simulink model "DMC"  (R2015b)
settings: Solver=VariableStepAuto  StartTime=0.0  StopTime=10.0  RelTol=1e-3
values from neighbouring files (symbols this model uses):
  b = 0.3    [demo_DMC.m]
  m = 1    [demo_DMC.m]
libraries: simulink x2
settings Model: Creator=mgreiff  LastModifiedBy=mgreiff

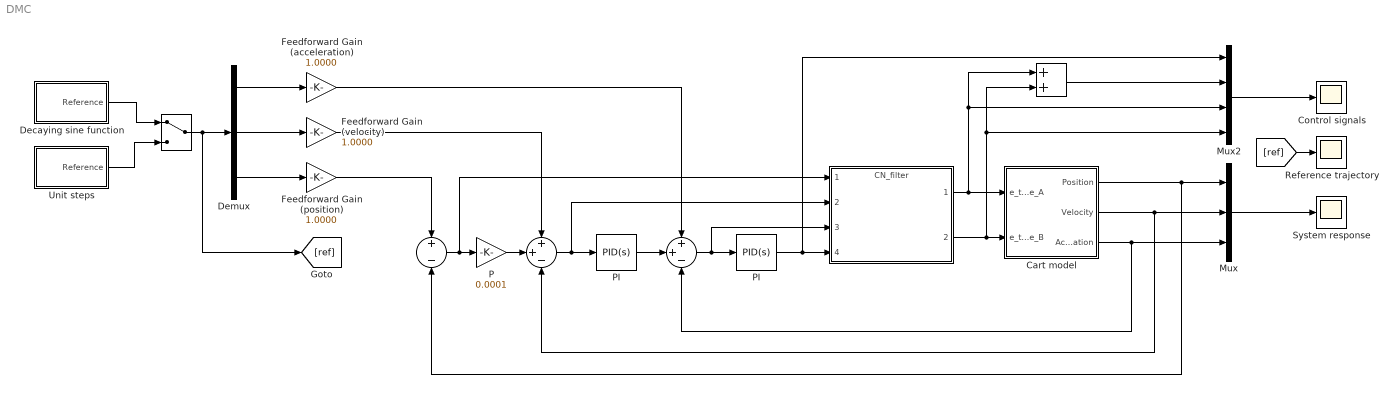
== system DMC ==
  " " : ModelReference  ModelNameDialog=CN_filter.slx  SimulationMode=Normal  ModelReferenceVersion=1.9  CopyOfModelName=CN_filter.slx
  "  " : Sum
  "   " : ManualSwitch
  "        " : Sum  Inputs=++-
  "         " : Sum  Inputs=++-
  "           " : Sum  Inputs=+|-
  "  PI    " : simulink/Continuous/PID Controller  Controller=PID  TimeDomain=Continuous-time  SampleTime=-1  IntegratorMethod=Forward Euler  FilterMethod=Forward Euler  Form=Parallel  UseFilter=on  ControllerParametersSource=internal  P=5  I=0.1  D=0  N=100  InitialConditionSource=internal  InitialConditionForIntegrator=0  InitialConditionForFilter=0  ExternalReset=none  LimitOutput=off  UpperSaturationLimit=inf  LowerSaturationLimit=-inf  LinearizeAsGain=on  AntiWindupMode=none  Kb=1  TrackingMode=off  Kt=1  PParamMin=[]  PParamMax=[]  IParamMin=[]  IParamMax=[]  DParamMin=[]  DParamMax=[]  NParamMin=[]  NParamMax=[]  KbParamMin=[]  KbParamMax=[]  KtParamMin=[]  KtParamMax=[]  POutMin=[]  POutMax=[]  IOutMin=[]  IOutMax=[]  DOutMin=[]  DOutMax=[]  NOutMin=[]  NOutMax=[]  KbOutMin=[]  KbOutMax=[]  KtOutMin=[]  KtOutMax=[]  IntegratorOutMin=[]  IntegratorOutMax=[]  FilterOutMin=[]  FilterOutMax=[]  SumOutMin=[]  SumOutMax=[]  SumI1OutMin=[]  SumI1OutMax=[]  SumI2OutMin=[]  SumI2OutMax=[]  SumI3OutMin=[]  SumI3OutMax=[]  SumDOutMin=[]  SumDOutMax=[]  SaturationOutMin=[]  SaturationOutMax=[]  IntegratorContinuousStateAttributes=''  IntegratorStateMustResolveToSignalObject=off  IntegratorRTWStateStorageClass=Auto  FilterContinuousStateAttributes=''  FilterStateMustResolveToSignalObject=off  FilterRTWStateStorageClass=Auto  DifferentiatorICPrevScaledInput=0  DifferentiatorOutMin=[]  DifferentiatorOutMax=[]
  Cart model : Subsystem
  Control signals : Scope
  Decaying sine function : Subsystem
  Demux : Demux  Outputs=3
  Feedforward Gain (acceleration) : Gain  Gain=1.0000
  Feedforward Gain (position) : Gain  Gain=1.0000
  Feedforward Gain (velocity) : Gain  Gain=1.0000
  Mux : Mux  Inputs=3
  Mux2 : Mux
  P : Gain  Gain=0.0001
  PI : simulink/Continuous/PID Controller  Controller=PID  TimeDomain=Continuous-time  SampleTime=-1  IntegratorMethod=Forward Euler  FilterMethod=Forward Euler  Form=Parallel  UseFilter=on  ControllerParametersSource=internal  P=4  I=0.1  D=0  N=100  InitialConditionSource=internal  InitialConditionForIntegrator=0  InitialConditionForFilter=0  ExternalReset=none  LimitOutput=off  UpperSaturationLimit=inf  LowerSaturationLimit=-inf  LinearizeAsGain=on  AntiWindupMode=none  Kb=1  TrackingMode=off  Kt=1  PParamMin=[]  PParamMax=[]  IParamMin=[]  IParamMax=[]  DParamMin=[]  DParamMax=[]  NParamMin=[]  NParamMax=[]  KbParamMin=[]  KbParamMax=[]  KtParamMin=[]  KtParamMax=[]  POutMin=[]  POutMax=[]  IOutMin=[]  IOutMax=[]  DOutMin=[]  DOutMax=[]  NOutMin=[]  NOutMax=[]  KbOutMin=[]  KbOutMax=[]  KtOutMin=[]  KtOutMax=[]  IntegratorOutMin=[]  IntegratorOutMax=[]  FilterOutMin=[]  FilterOutMax=[]  SumOutMin=[]  SumOutMax=[]  SumI1OutMin=[]  SumI1OutMax=[]  SumI2OutMin=[]  SumI2OutMax=[]  SumI3OutMin=[]  SumI3OutMax=[]  SumDOutMin=[]  SumDOutMax=[]  SaturationOutMin=[]  SaturationOutMax=[]  IntegratorContinuousStateAttributes=''  IntegratorStateMustResolveToSignalObject=off  IntegratorRTWStateStorageClass=Auto  FilterContinuousStateAttributes=''  FilterStateMustResolveToSignalObject=off  FilterRTWStateStorageClass=Auto  DifferentiatorICPrevScaledInput=0  DifferentiatorOutMin=[]  DifferentiatorOutMax=[]
  Reference trajectory : Scope
  System response : Scope
  Unit steps : Subsystem
  wires:
  Cart model/1(Position) -> Mux/1, "           "/2
  Cart model/2(Velocity) -> "        "/3, Mux/2
  " "/1 -> "  "/1, Mux2/3, Cart model/1(e_torque_A)
  " "/2 -> "  "/2, Mux2/4, Cart model/2(e_torque_B)
  "   "/1 -> [ref], Demux/1
  Demux/3 -> Feedforward Gain (position)/1
  "           "/1 -> " "/1, P/1
  P/1 -> "        "/2
  "        "/1 -> "  PI    "/1, " "/2
  "         "/1 -> " "/3, PI/1
  "  PI    "/1 -> "         "/2
  Cart model/3(Acceleration) -> "         "/3, Mux/3
  Demux/2 -> Feedforward Gain (velocity)/1
  Demux/1 -> Feedforward Gain (acceleration)/1
  PI/1 -> Mux2/1, " "/4
  Mux/1 -> System response/1
  Unit steps/1(Reference) -> "   "/2
  Decaying sine function/1(Reference) -> "   "/1
  Mux2/1 -> Control signals/1
  Feedforward Gain (acceleration)/1 -> "         "/1
  Feedforward Gain (velocity)/1 -> "        "/1
  Feedforward Gain (position)/1 -> "           "/1
  "  "/1 -> Mux2/2
  [ref] -> Reference trajectory/1

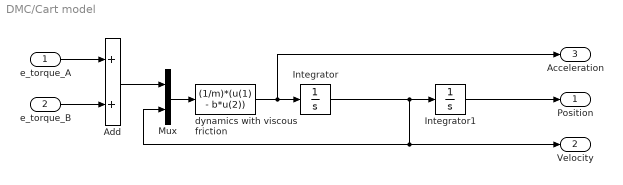
== system DMC/Cart model ==
  e_torque_A : Inport
  e_torque_B : Inport  Port=2
  Add : Sum
  Integrator : Integrator
  Integrator1 : Integrator
  Mux : Mux  Inputs=2
  dynamics with viscous friction : Fcn  Expr=(1/m)*(u(1) - b*u(2))
  Position : Outport
  Velocity : Outport  Port=2
  Acceleration : Outport  Port=3
  wires:
  Mux/1 -> dynamics with viscous friction/1
  dynamics with viscous friction/1 -> Acceleration/1, Integrator/1
  e_torque_B/1 -> Add/2
  Integrator1/1 -> Position/1
  Integrator/1 -> Mux/2, Velocity/1, Integrator1/1
  e_torque_A/1 -> Add/1
  Add/1 -> Mux/1

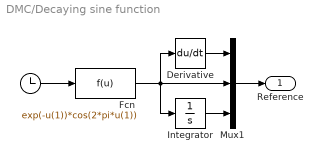
== system DMC/Decaying sine function ==
  "  " : Clock
  Derivative : Derivative
  Fcn : Fcn  Expr=exp(-u(1))*cos(2*pi*u(1))
  Integrator : Integrator
  Mux1 : Mux  Inputs=3
  Reference : Outport
  wires:
  "  "/1 -> Fcn/1
  Derivative/1 -> Mux1/1
  Fcn/1 -> Integrator/1, Derivative/1, Mux1/2
  Mux1/1 -> Reference/1
  Integrator/1 -> Mux1/3

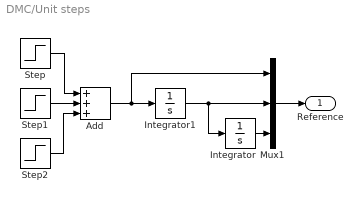
== system DMC/Unit steps ==
  Add : Sum  Inputs=+++
  Integrator : Integrator
  Integrator1 : Integrator
  Mux1 : Mux  Inputs=3
  Step : Step  Time=2  After=2  SampleTime=0
  Step1 : Step  Time=4  After=-4  SampleTime=0
  Step2 : Step  Time=6  After=2  SampleTime=0
  Reference : Outport
  wires:
  Add/1 -> Integrator1/1, Mux1/1
  Mux1/1 -> Reference/1
  Integrator/1 -> Mux1/3
  Integrator1/1 -> Mux1/2, Integrator/1
  Step/1 -> Add/1
  Step1/1 -> Add/2
  Step2/1 -> Add/3
